simulink model "model2"  (R2021a)
settings: Solver=VariableStepAuto  StartTime=0.0  StopTime=10.0  RelTol=1e-3
model workspace (MAT data in the model file):
  K = -9.2
undefined symbols (not defined in the file): Ion, Lithium
libraries: spsGroundLib x2, spsBatteryLib x1, spsControlledCurrentSourceLib x1, fuzblock x1, spspowerguiLib x1
settings Model: Creator=Sreedhar  LastModifiedBy=Sreedhar

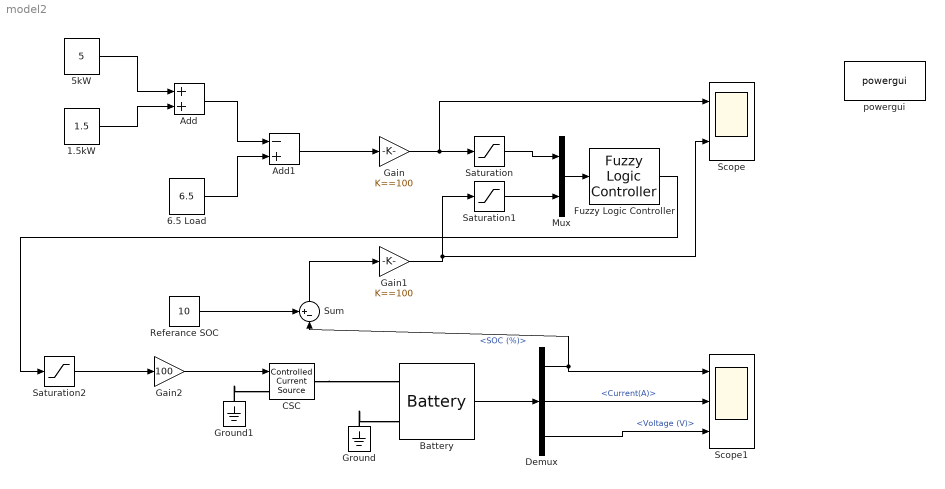
== system model2 ==
  1.5kW : Constant  Value=1.5
  5kW : Constant  Value=5
  6.5 Load : Constant  Value=6.5
  Add : Sum
  Add1 : Sum  Inputs=-+
  Battery : spsBatteryLib/Battery  BatType=Lithium-Ion  ShowTempParam=off  ThermalPreset="3.6V  3.6Ah  (LiNiO2)"  ShowAgeParam=on  NomV=3.1  NomQ=3.6  SOC=100  Batt_Tr=30  PresetModel=off  MaxQ=3.2  MinV=2.325  FullV=3.75  Dis_rate=0.72  R=0.00889  Normal_OP=2.8  expZone="[3.5         0.5]"  current=[6.5 13 32.5]  Units=Time  Tci=20  NomT=20  T2=0  MaxQ2=2.7  FullV2=3.5  Normal_OP2=2.94  expZone2="[3.25         0.5]"  Rca=0.6  ti=1000  Dp=0  Neq0=0  Tsim=1e6  Ta1=25  Qeol=5.4*0.9  Reol=0.013333*1.2  Char_age=[2.3478, 3]  Dis_age=[2.3478, 10]  N1=1500  N2=10500  N3=1000  N4=1400  Ta2=45  N5=950
  CSC : spsControlledCurrentSourceLib/Controlled Current Source  Initialize=on  Source_Type=AC  Amplitude=100  Phase=0  Frequency=50  Measurements=Current
  Demux : Demux  Outputs=3
  Fuzzy Logic Controller : fuzblock/Fuzzy Logic  Controller  FIS='Fuzzymain.fis'  OutputSampleNumber=101  DataType=double  FuzzifiedInputs=off  RuleFiringStrengths=off  RuleOutputs=off  AggregatedOutputs=off  SimulateUsing=Code generation  OutOfRangeInputValueMessage=warning  NoRuleFiredMessage=warning  EmptyOutputFuzzySetMessage=warning
  Gain : Gain  Gain=K==100
  Gain1 : Gain  Gain=K==100
  Gain2 : Gain  Gain=100
  Ground : spsGroundLib/Ground  LConnTagsString=a
  Ground1 : spsGroundLib/Ground  LConnTagsString=a
  Mux : Mux  Inputs=2
  Referance SOC : Constant  Value=10
  Saturation : Saturate  LinearizeAsGain=off  ZeroCross=off
  Saturation1 : Saturate  LinearizeAsGain=off  ZeroCross=off
  Saturation2 : Saturate  LinearizeAsGain=off  ZeroCross=off
  Scope : Scope  NumInputPorts=2
  Scope1 : Scope  NumInputPorts=3
  Sum : Sum  Inputs=+-|
  powergui : spspowerguiLib/powergui  Priority=1  SimulationMode=Discrete  SampleTime=50e-6  frequency=60  Iterations=50  frequencyindice=0  Pbase=100e6  ErrMax=1e-4  UnitsV=kV  UnitsW=MW  buscounter=0  FunctionMessages=off  echomessages=off  EnableUseOfTLC=off  CurrentSourceSwitches=off  DisableSnubberDevices=off  DisableRonSwitches=off  DisableVfSwitches=off  DisplayEquations=off  AutomaticDiscreteSolvers=off  SolverType=Tustin/Backward Euler (TBE)  Interpol=off  ExternalGateDelay=off  methode=off  Ts=100  x0status=blocks  SPID=on  SwTol=0  HookPort=off  NonlinearTolerance=1e-4  nMaxIteration=100  ContinueOnMaxIteration=off  RestoreLinks=warning  ResistiveCurrentMeasurement=off  Frange=[0:2:500]  Ylog=off  Xlog=on  ShowGrid=off  save=off  variable=ZData  structure=0  ZoomFFT=off  StartTime=0.0  cycles=1  DisplayStyle=1  fundamental=60  FreqAxis=off  MaxFrequency=1000  frequencyindicesteady=1  RmsSteady=1  display=off
  wires:
  5kW/1 -> Add/1
  1.5kW/1 -> Add/2
  Add/1 -> Add1/1
  6.5 Load/1 -> Add1/2
  Add1/1 -> Gain/1
  Gain/1 -> Scope/1, Saturation/1
  Saturation/1 -> Mux/1
  Saturation1/1 -> Mux/2
  Mux/1 -> Fuzzy Logic Controller/1
  Gain1/1 -> Scope/2, Saturation1/1
  Sum/1 -> Gain1/1
  Referance SOC/1 -> Sum/1
  Saturation2/1 -> Gain2/1
  Gain2/1 -> CSC/1
  Battery/1 -> Demux/1
  Demux/1 -> Scope1/1, Sum/2  "<SOC (%)>"
  Demux/2 -> Scope1/2  "<Current(A)>"
  Demux/3 -> Scope1/3  "<Voltage (V)>"
  Fuzzy Logic Controller/1 -> Saturation2/1
  connections:
  CSC/RConn1 -- Battery/LConn2
  Ground/LConn1 -- Battery/LConn1
  Ground1/LConn1 -- CSC/LConn1
